simulink model "task16_8"  (R2021a)
settings: Solver=VariableStepAuto  StartTime=0.0  StopTime=10.0  RelTol=1e-3
settings Model: Creator=reemb  LastModifiedBy=reemb

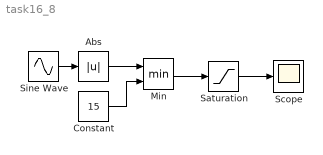
== system task16_8 ==
  Abs : Abs
  Constant : Constant  Value=15
  Min : MinMax  Inputs=2
  Saturation : Saturate  UpperLimit=10  LowerLimit=5
  Scope : Scope
  Sine Wave : Sin  Amplitude=20  SampleTime=0
  wires:
  Sine Wave/1 -> Abs/1
  Abs/1 -> Min/1
  Constant/1 -> Min/2
  Saturation/1 -> Scope/1
  Min/1 -> Saturation/1
